simulink model "Fuzzy_3"  (R2015b)
settings: Solver=ode8  StartTime=0.0  StopTime=20  FixedStep=0.0001  RelTol=1e-3
libraries: fuzblock x2
settings Model: Creator=jalili  LastModifiedBy=jalili

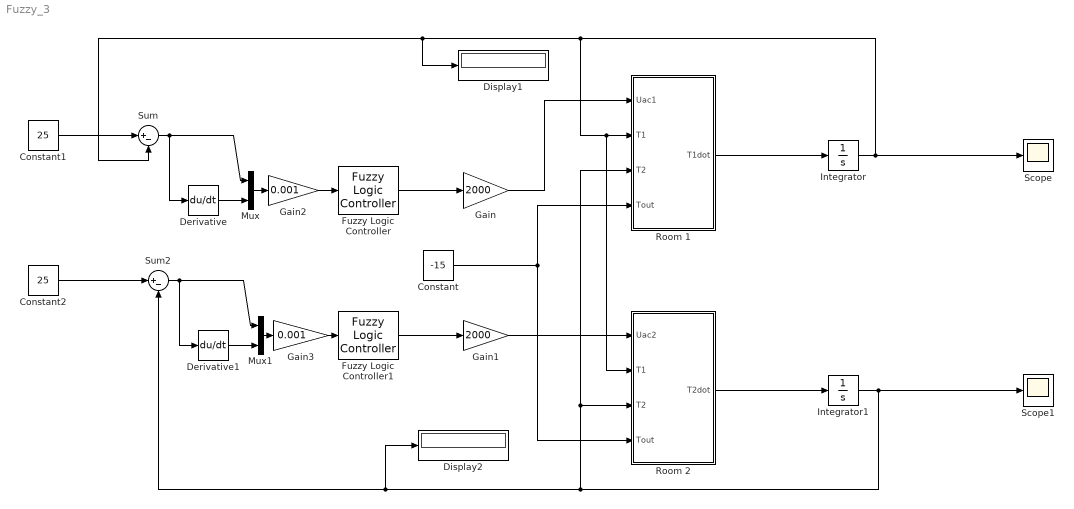
== system Fuzzy_3 ==
  Constant : Constant  Value=-15
  Constant1 : Constant  Value=25
  Constant2 : Constant  Value=25
  Derivative : Derivative
  Derivative1 : Derivative
  Display1 : Display
  Display2 : Display
      settings: Decimation=100
  Fuzzy Logic Controller : fuzblock/Fuzzy Logic  Controller  fis='fuzzy.fis'
  Fuzzy Logic Controller1 : fuzblock/Fuzzy Logic  Controller  fis='fuzzy.fis'
  Gain : Gain  Gain=2000
  Gain1 : Gain  Gain=2000
  Gain2 : Gain  Gain=0.001
  Gain3 : Gain  Gain=0.001
  Integrator : Integrator  InitialCondition=30
  Integrator1 : Integrator  InitialCondition=27
  Mux : Mux  Inputs=2
  Mux1 : Mux  Inputs=2
  Room 1 : MATLAB Function  TreatAsAtomicUnit=on
  Room 2 : MATLAB Function  TreatAsAtomicUnit=on
  Scope : Scope
  Scope1 : Scope
  Sum : Sum  Inputs=|+-
  Sum2 : Sum  Inputs=|+-
  wires:
  Room 1/1(T1dot) -> Integrator/1
  Room 2/1(T2dot) -> Integrator1/1
  Integrator1/1 -> Scope1/1, Display2/1, Sum2/2, Room 1/3(T2), Room 2/3(T2)
  Integrator/1 -> Scope/1, Room 2/2(T1), Room 1/2(T1), Display1/1, Sum/2
  Constant/1 -> Room 2/4(Tout), Room 1/4(Tout)
  Mux/1 -> Gain2/1
  Sum/1 -> Derivative/1, Mux/1
  Constant1/1 -> Sum/1
  Derivative/1 -> Mux/2
  Sum2/1 -> Derivative1/1, Mux1/1
  Derivative1/1 -> Mux1/2
  Mux1/1 -> Gain3/1
  Fuzzy Logic Controller/1 -> Gain/1
  Gain/1 -> Room 1/1(Uac1)
  Fuzzy Logic Controller1/1 -> Gain1/1
  Gain1/1 -> Room 2/1(Uac2)
  Gain2/1 -> Fuzzy Logic Controller/1
  Gain3/1 -> Fuzzy Logic Controller1/1
  Constant2/1 -> Sum2/1

== matlab function Fuzzy_3/Room 2 ==
  data: Uac2 input; T2dot output; T1 input; T2 input; Tout input
function T2dot = fcn(Uac2, T1, T2, Tout)
T2dot = -0.039 * T2 + 0.01 * T1 + 0.0075 * Tout + Uac2;

== matlab function Fuzzy_3/Room 1 ==
  data: Uac1 input; T1dot output; T1 input; T2 input; Tout input
function T1dot = fcn(Uac1, T1, T2, Tout)
T1dot = -0.05 * T1 + 0.01 * T2 + 0.008 * Tout + Uac1;
